simulink model "sim_controladores"  (R2025a)
settings: Solver=FixedStepAuto  StartTime=0.0  StopTime=30.0  RelTol=1e-3
values from neighbouring files (symbols this model uses):
  a = 0.049017947318623 / 1.047866225848407    (= 0.0467788216754)    [diseno_controladores.m]
  K = 0.920379287458449    (= 0.920379287458)    [diseno_controladores.m]    (also in orden1_controladores.m = 0.92044)
  Kp = (2*xi_m*Tm1)/(K*L) * (1 - 1/Ms)    [diseno_controladores.m]    (also in orden1_controladores.m = (T + 0.5*L) / (K * (lambda + L)))
  L = 0.089649500000000    (= 0.0896495)    [diseno_controladores.m]    (also in orden1_controladores.m = 0.1371)
  T = 1.047866225848407    (= 1.04786622585)    [diseno_controladores.m]    (also in orden1_controladores.m = 1.0507)
  Td = Tm1/(2*xi_m)    [diseno_controladores.m]    (also in orden1_controladores.m = 0.0643515613134)
  Ti = 2*xi_m*Tm1    [diseno_controladores.m]    (also in orden1_controladores.m = 1.11925)
settings Model: Creator=danielsaenzobando  LastModifiedBy=danielsaenzobando

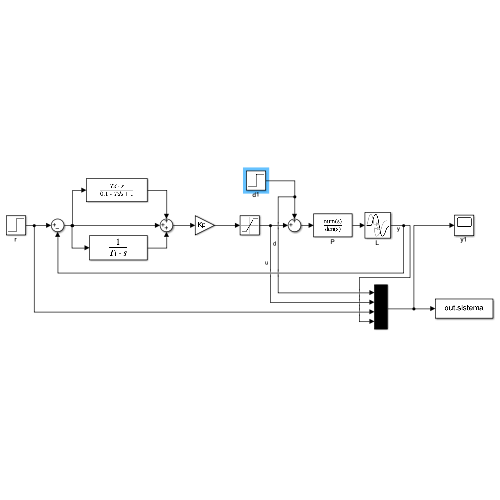
[thumbnail: Simulink's stored preview of the top-level diagram]
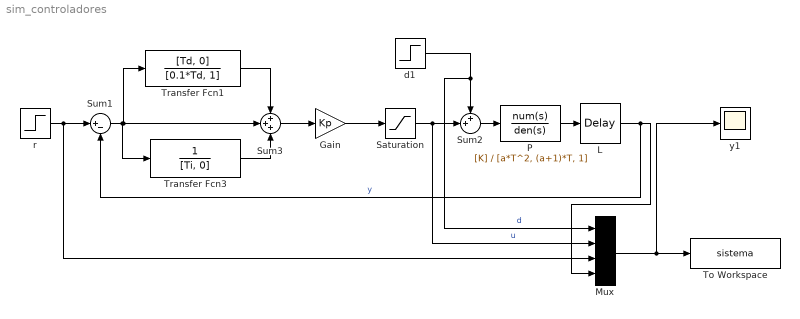
== system sim_controladores ==
  Gain : Gain  Gain=Kp
  L : TransportDelay  DelayTime=L
  Mux : Mux
  P : TransferFcn  Numerator=[K]  Denominator=[a*T^2, (a+1)*T, 1]
  Saturation : Saturate  UpperLimit=100  LowerLimit=0
  Sum1 : Sum  Inputs=|+-
  Sum2 : Sum  Inputs=++|
  Sum3 : Sum  Inputs=+++
  To Workspace : ToWorkspace  VariableName=sistema  SaveFormat=Timeseries  SampleTime=-1
  Transfer Fcn1 : TransferFcn  Numerator=[Td, 0]  Denominator=[0.1*Td, 1]
  Transfer Fcn3 : TransferFcn  Denominator=[Ti, 0]
  d1 : Step  Time=15  After=10  SampleTime=0
  "r " : Step  Time=5  After=20  SampleTime=0
  y1 : Scope
      settings: ActiveDisplayYMinimum=-39.063047037354828  ActiveDisplayYMaximum=135.53887336337169
  wires:
  Sum2/1 -> P/1
  Mux/1 -> y1/1, To Workspace/1
  L/1 -> Mux/4, Sum1/2  "y"
  "r "/1 -> Mux/3, Sum1/1
  Sum1/1 -> Sum3/2, Transfer Fcn1/1, Transfer Fcn3/1
  P/1 -> L/1
  Gain/1 -> Saturation/1
  Sum3/1 -> Gain/1
  Transfer Fcn1/1 -> Sum3/1
  Transfer Fcn3/1 -> Sum3/3
  Saturation/1 -> Sum2/2, Mux/2  "u"
  d1/1 -> Sum2/1, Mux/1  "d"
